simulink model "DynamixelLibrary_Prototyping"  (R2017b)
settings: Solver=FixedStepAuto  StartTime=0.0  StopTime=10  FixedStep=0.05  RelTol=1e-3  EnableMultiTasking=on
settings Model: SimulationMode=external  Creator=AlexC  LastModifiedBy=SRCL
settings SolverCC: PositivePriorityOrder=on
settings OptimizationCC: PassReuseOutputArgsThreshold=0  MaxStackSize=64
settings DebuggingCC: ParameterTunabilityLossMsg=error
settings HardwareCC: ProdBitPerPointer=32  ProdBitPerSizeT=32  ProdBitPerPtrDiffT=32  ProdLargestAtomicInteger=Long  ProdLargestAtomicFloat=Double  ProdWordSize=32  ProdHWDeviceType=ARM Compatible->ARM Cortex
settings SFSimCC: MATLABDynamicMemAlloc=off
settings RTWCC: SystemTargetFile=ert.tlc  HardwareBoard=Raspberry Pi  TemplateMakefile=ert_default_tmf  Toolchain=GNU GCC Raspberry Pi  BuildConfiguration=Specify  TargetLang=C++
settings CodeAppCC: ForceParamTrailComments=on  OperatorAnnotations=on
settings ERTTargetCC: CodeReplacementLibrary=GCC ARM Cortex-A8  ERTCustomFileBanners=off  SupportContinuousTime=on  SupportNonInlinedSFcns=on  RemoveResetFunc=off  SupportVariableSizeSignals=on  ModelStepFunctionPrototypeControlCompliant=off  RootIOFormat=Structure reference

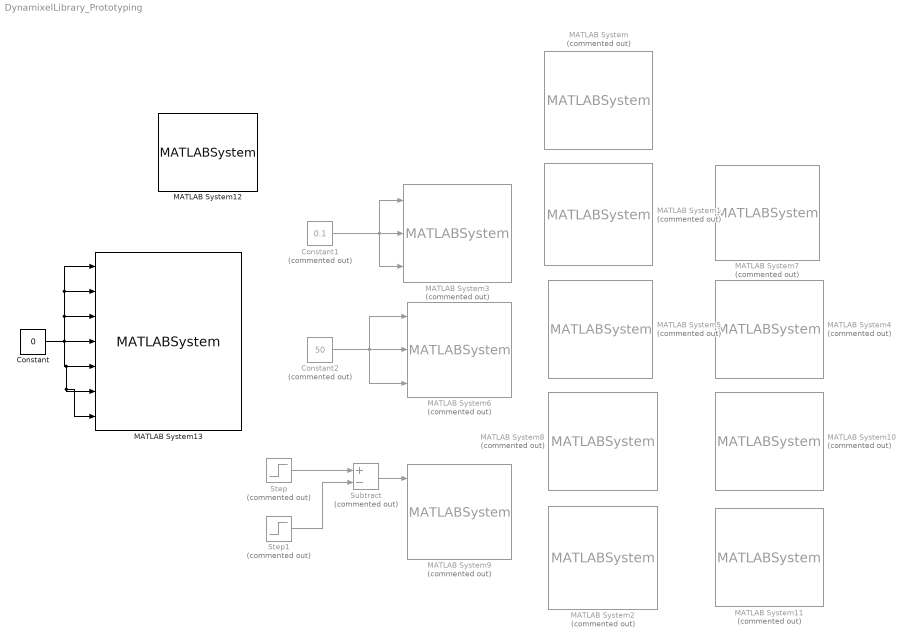
== system DynamixelLibrary_Prototyping ==
  Constant : Constant  Value=0
  Constant1 : Constant  Commented=on  Value=0.1
  Constant2 : Constant  Commented=on  Value=50
  MATLAB System : MATLABSystem  Commented=on  System=InitializeForPosition  P_GAIN=400  I_GAIN=0  D_GAIN=200  MAX_POSITION=3072  MIN_POSITION=1024  VELOCITY_LIMIT=100
      mask Type: InitializeForPosition
      mask Display: disp('InitializeForPosition');
  MATLAB System1 : MATLABSystem  Commented=on  System=InitializeForSpeed  P_GAIN=100  I_GAIN=1920  VELOCITY_LIMIT=1023
      mask Type: InitializeForSpeed
      mask Display: disp('InitializeForSpeed');
  MATLAB System10 : MATLABSystem  Commented=on  System=InitializeForSpecial  CURRENT_LIMIT=850  P_GAIN=400  I_GAIN=0  D_GAIN=200  MAX_POSITION=3072  MIN_POSITION=1024  VELOCITY_LIMIT=0
      mask Type: InitializeForSpecial
      mask Display: disp('InitializeForSpecial');
  MATLAB System11 : MATLABSystem  Commented=on  System=MoveArm_Special
      mask Type: MoveArm_Special
      mask Display:
      | disp('MoveArm_Special');
      | port_label('input',1,'u1');
      | port_label('input',2,'u2');
      | port_label('input',3,'u3');
  MATLAB System12 : MATLABSystem  System=InitializeForArmGripper  P_GAIN_ARM=400  I_GAIN_ARM=0  D_GAIN_ARM=200  P_GAIN_PROX=400  I_GAIN_PROX=0  D_GAIN_PROX=200  P_GAIN_DIST=400  I_GAIN_DIST=0  D_GAIN_DIST=200  MAX_POSITION_ARM=3072  MIN_POSITION_ARM=1024  MAX_POSITION_PROX=3072  MIN_POSITION_PROX=1024  MAX_POSITION_DIST=3072  MIN_POSITION_DIST=1024  VELOCITY_LIMIT_ARM=0  VELOCITY_LIMIT_GRIP=0  MAX_CURRENT_GRIP=1000
      mask Type: InitializeForArmGripper
      mask Display: disp('InitializeForArmGripper');
  MATLAB System13 : MATLABSystem  System=MoveArmGripper_Position
      mask Type: MoveArmGripper_Position
      mask Display:
      | disp('MoveArmGripper_Position');
      | port_label('input',1,'u1');
      | port_label('input',2,'u2');
      | port_label('input',3,'u3');
      | port_label('input',4,'uL1');
      | port_label('input',5,'uR1');
      | port_label('input',6,'uL2');
      | port_label('input',7,'uR2');
  MATLAB System2 : MATLABSystem  Commented=on  System=MoveArm_Position
      mask Type: MoveArm_Position
      mask Display:
      | disp('MoveArm_Position');
      | port_label('input',1,'u1');
      | port_label('input',2,'u2');
      | port_label('input',3,'u3');
  MATLAB System3 : MATLABSystem  Commented=on  System=MoveArm_Speed
      mask Type: MoveArm_Speed
      mask Display:
      | disp('MoveArm_Speed');
      | port_label('input',1,'u1');
      | port_label('input',2,'u2');
      | port_label('input',3,'u3');
  MATLAB System4 : MATLABSystem  Commented=on  System=ReadArm_Position  SampleTime=0.05
      mask Type: ReadArm_Position
      mask Display:
      | disp('ReadArm_Position');
      | port_label('output',1,'y1');
      | port_label('output',2,'y2');
      | port_label('output',3,'y3');
  MATLAB System5 : MATLABSystem  Commented=on  System=InitializeForPWM  PWM_LIMIT=885
      mask Type: InitializeForPWM
      mask Display: disp('InitializeForPWM');
  MATLAB System6 : MATLABSystem  Commented=on  System=MoveArm_PWM
      mask Type: MoveArm_PWM
      mask Display:
      | disp('MoveArm_PWM');
      | port_label('input',1,'u1');
      | port_label('input',2,'u2');
      | port_label('input',3,'u3');
  MATLAB System7 : MATLABSystem  Commented=on  System=ReadArm_Load  SampleTime=0.1
      mask Type: ReadArm_Load
      mask Display:
      | disp('ReadArm_Load');
      | port_label('output',1,'y1');
      | port_label('output',2,'y2');
      | port_label('output',3,'y3');
  MATLAB System8 : MATLABSystem  Commented=on  System=InitializeForTorque  CURRENT_LIMIT=850
      mask Type: InitializeForTorque
      mask Display: disp('InitializeForTorque');
  MATLAB System9 : MATLABSystem  Commented=on  System=MoveArm_Torque
      mask Type: MoveArm_Torque
      mask Display:
      | disp('MoveArm_Torque');
      | port_label('input',1,'u1');
      | port_label('input',2,'u2');
      | port_label('input',3,'u3');
      | port_label('output',1,'y1');
      | port_label('output',2,'y2');
      | port_label('output',3,'y3');
  Step : Step  Commented=on  Time=5  After=30  SampleTime=0
  Step1 : Step  Commented=on  Time=6  After=30  SampleTime=0
  Subtract : Sum  Commented=on  Inputs=+-
  wires:
  Constant1/1 -> MATLAB System3/1, MATLAB System3/3, MATLAB System3/2
  Constant2/1 -> MATLAB System6/3, MATLAB System6/1, MATLAB System6/2
  Step/1 -> Subtract/1
  Step1/1 -> Subtract/2
  Subtract/1 -> MATLAB System9/1
  Constant/1 -> MATLAB System13/7, MATLAB System13/6, MATLAB System13/5, MATLAB System13/3, MATLAB System13/2, MATLAB System13/1, MATLAB System13/4
